simulink model "PD_point2point"  (R2019b)
settings: Solver=VariableStepAuto  StartTime=0.0  StopTime=10.0  RelTol=1e-3
values from neighbouring files (symbols this model uses):
  dq0 = (zeros(1,6))'    [initAdaptiveCompTorque.m]    (also in initCompTorque.m; initCompTorqueReg.m; initPD_traj.m)
  parameter = [d, m, theta0]    [init.m]    (also in initAdaptiveCompTorque.m = [parameter, theta0]; initCompTorque.m = [parameter, theta0]; initCompTorqueReg.m = [parameter, theta0]; initPD_traj.m = [parameter, theta0])
  q0 = q0 + delta    [initAdaptiveCompTorque.m]    (also in initCompTorque.m; initCompTorqueReg.m = [0 0 0 0 0 0]'; initPD_traj.m)
undefined symbols (not defined in the file or in its folder): xd
settings Model: Creator=giga4  LastModifiedBy=giga4

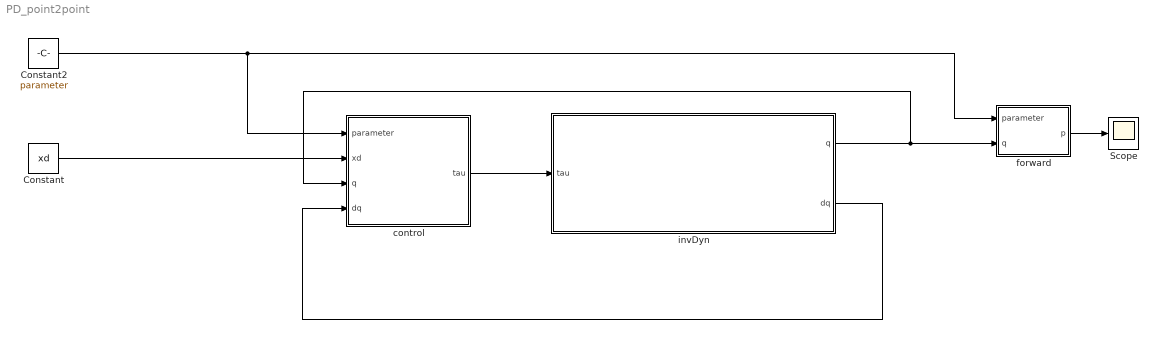
== system PD_point2point ==
  Constant : Constant  Value=xd
  Constant2 : Constant  Value=parameter
  Scope : Scope
  control : MATLAB Function  TreatAsAtomicUnit=on
  "forward " : MATLAB Function  TreatAsAtomicUnit=on
  "invDyn " : Subsystem
  wires:
  control/1(tau) -> "invDyn "/1(tau)
  "invDyn "/2(dq) -> control/4(dq)
  "invDyn "/1(q) -> "forward "/2(q), control/3(q)
  Constant/1 -> control/2(xd)
  Constant2/1 -> "forward "/1(parameter), control/1(parameter)
  "forward "/1(p) -> Scope/1

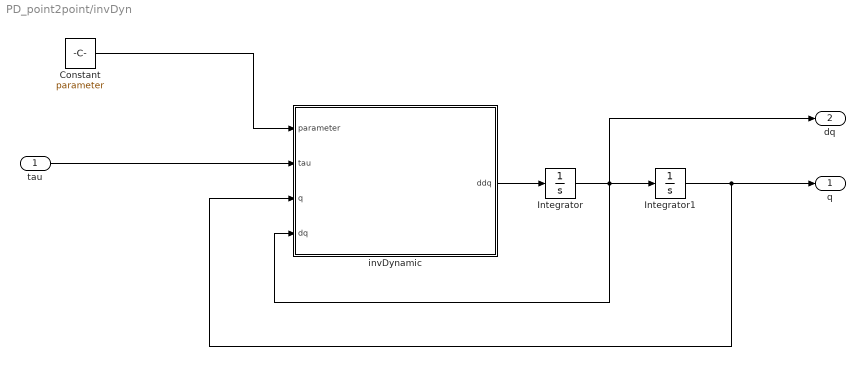
== system PD_point2point/invDyn  ==
  tau : Inport
  Constant : Constant  Value=parameter
  Integrator : Integrator  InitialCondition=dq0
  Integrator1 : Integrator  InitialCondition=q0
  "invDynamic " : MATLAB Function  TreatAsAtomicUnit=on
  q : Outport
  dq : Outport  Port=2
  wires:
  Integrator1/1 -> q/1, "invDynamic "/3(q)
  "invDynamic "/1(ddq) -> Integrator/1
  tau/1 -> "invDynamic "/2(tau)
  Constant/1 -> "invDynamic "/1(parameter)
  Integrator/1 -> Integrator1/1, dq/1, "invDynamic "/4(dq)

== matlab function PD_point2point/control ==
  data: parameter input; xd input; q input; tau output; dq input
function tau = control(parameter, xd, q,dq)

    J = J_end_f(parameter,q,dq);
    Jp = J(1:3,:);  %%SOLO QUELLE RELATIVe alla pos
    
    G = G_f(parameter,q,dq);
    p_now = forwardKinematics(parameter, q);
    Kv = 100*eye(6);
    K = eye(3);
    JpK = (Jp')*K;
    e = (xd - p_now(1:3,4));
    
    tau = JpK*e - Kv*dq - G;

end

== matlab function PD_point2point/invDyn /invDynamic  ==
  data: parameter input; tau input; ddq output; q input; dq input
function ddq = inverseDynamic(parameter,tau,q,dq)

    B = B_f(parameter,q,dq);
    C = C_f(parameter,q,dq); 
    G = G_f(parameter,q,dq);

    ddq = B\(tau-C*dq-G);

== matlab function PD_point2point/forward  ==
  data: parameter input; q input; p output
function p = forwardKine(parameter, q)

    [Etip,T00,T01,T12,T23,T34,T45,T56] = forwardKinematics(parameter, q);

    p = Etip(1:3,4);
